simulink model "SpeedPLL"  (R2019b)
settings: Solver=VariableStepAuto  StartTime=0.0  StopTime=1  MaxStep=1/15000  MinStep=0.99/15000
libraries: simulink x1
settings Model: Creator=lenovo  LastModifiedBy=lenovo

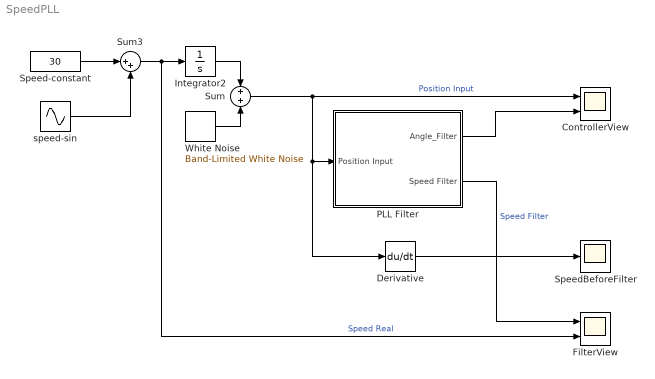
== system SpeedPLL ==
  ControllerView : Scope  NumInputPorts=2
  Derivative : Derivative
  FilterView : Scope  NumInputPorts=2
  Integrator2 : Integrator
  PLL Filter : Subsystem
  Speed-constant : Constant  Value=30
  SpeedBeforeFilter : Scope
  Sum : Sum  Inputs=+|+
  Sum3 : Sum  Inputs=|++
  White Noise : simulink/Sources/Band-Limited White Noise  Cov=0.0000005  Ts=1/1000  seed=[23341]
  speed-sin : Sin  Amplitude=10  Frequency=2*2*pi  SampleTime=0
  wires:
  Integrator2/1 -> Sum/1
  Sum/1 -> Derivative/1, PLL Filter/1(Position Input), ControllerView/1  "Position Input"
  Derivative/1 -> SpeedBeforeFilter/1
  White Noise/1 -> Sum/2
  speed-sin/1 -> Sum3/2
  Speed-constant/1 -> Sum3/1
  Sum3/1 -> FilterView/2, Integrator2/1  "Speed Real"
  PLL Filter/1(Angle_Filter) -> ControllerView/2
  PLL Filter/2(Speed Filter) -> FilterView/1  "Speed Filter"

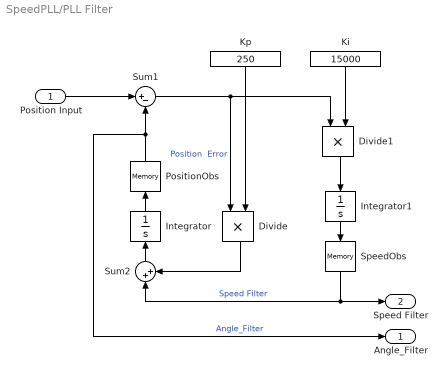
== system SpeedPLL/PLL Filter ==
  Position Input : Inport
  Divide : Product  Inputs=**
  Divide1 : Product  Inputs=**
  Integrator : Integrator
  Integrator1 : Integrator
  Ki : Constant  Value=15000
  Kp : Constant  Value=250
  PositionObs : Memory  StateName=ThetaObs
  SpeedObs : Memory  StateName=SpeedObs
  Sum1 : Sum  Inputs=|+-
  Sum2 : Sum  Inputs=|++
  Angle_Filter : Outport
  Speed Filter : Outport  Port=2
  wires:
  PositionObs/1 -> Sum1/2, Angle_Filter/1  "Angle_Filter"
  Position Input/1 -> Sum1/1
  Integrator/1 -> PositionObs/1
  SpeedObs/1 -> Sum2/1, Speed Filter/1  "Speed Filter"
  Kp/1 -> Divide/2
  Integrator1/1 -> SpeedObs/1
  Divide1/1 -> Integrator1/1
  Divide/1 -> Sum2/2
  Sum2/1 -> Integrator/1
  Ki/1 -> Divide1/2
  Sum1/1 -> Divide1/1, Divide/1  "Position  Error"
